simulink model "ARM_Open_loop_simulation"  (R2021a)
settings: Solver=VariableStepAuto  StartTime=0.0  StopTime=50  RelTol=1e-3  EnableMultiTasking=on
StartFcn:
  | clear all
libraries: simulink x1, realtime_pacer_lib x1
settings Model: Creator=johnh  LastModifiedBy=Andy
settings SolverCC: AlgebraicLoopSolver=TrustRegion
settings DataIOCC: ReturnWorkspaceOutputs=off
settings OptimizationCC: LifeSpan=inf
settings DebuggingCC: SFUnexpectedBacktrackingDiag=warning  SFNoUnconditionalDefaultTransitionDiag=warning  SFMachineParentedDataDiag=warning  ArithmeticOperatorsInVariantConditions=warning
settings SFSimCC: SimUseLocalCustomCode=off  CustomCodeUndefinedFunction=UseInterfaceOnly
settings RTWCC: RTWUseLocalCustomCode=off
settings CodeAppCC: StateflowObjectComments=on
settings GRTTargetCC: TargetLangStandard=C89/C90 (ANSI)
settings ConfigComp: CovMetricSettings=dw  CovSaveCumulativeToWorkspaceVar=on  CovSaveSingleToWorkspaceVar=on  CovExternalEMLEnable=off

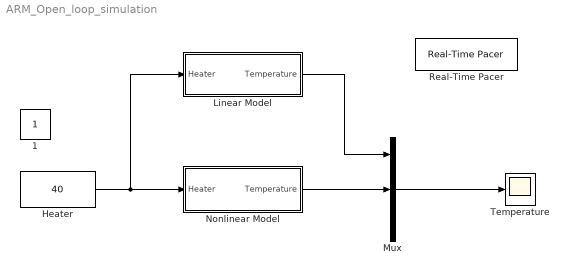
== system ARM_Open_loop_simulation ==
  Heater : simulink/Math Operations/Slider Gain  gain=40  low=0  high=100
  Linear Model : Subsystem
  Mux : Mux  Inputs=3
  Nonlinear Model : Subsystem
  Real-Time Pacer : realtime_pacer_lib/Real-Time Pacer  simTimePerRealTime=1
  Temperature : Scope
  1 : Constant  IOType=siggen
  wires:
  Mux/1 -> Temperature/1
  Linear Model/1(Temperature) -> Mux/1
  Nonlinear Model/1(Temperature) -> Mux/2
  Heater/1 -> Linear Model/1(Heater), Nonlinear Model/1(Heater)

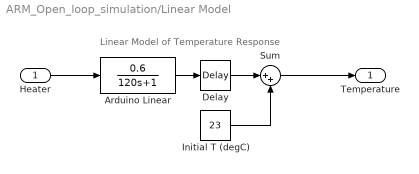
== system ARM_Open_loop_simulation/Linear Model ==
  note: Linear Model of Temperature Response
  Heater : Inport
  Arduino Linear : TransferFcn  Numerator=[0.6]  Denominator=[120 1]
  Delay : TransportDelay  DelayTime=3
  Initial T (degC) : Constant  Value=23
  Sum : Sum  Inputs=|++
  Temperature : Outport
  wires:
  Arduino Linear/1 -> Delay/1
  Delay/1 -> Sum/1
  Initial T (degC)/1 -> Sum/2
  Sum/1 -> Temperature/1
  Heater/1 -> Arduino Linear/1

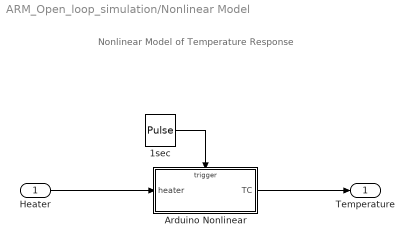
== system ARM_Open_loop_simulation/Nonlinear Model ==
  note: Nonlinear Model of Temperature Response
  Heater : Inport
  1sec : DiscretePulseGenerator  PulseType=Time based  Period=1  PulseWidth=50
  Arduino Nonlinear : Subsystem  TreatAsAtomicUnit=on
  Temperature : Outport
  wires:
  1sec/1 -> Arduino Nonlinear/Trigger
  Arduino Nonlinear/1(TC) -> Temperature/1
  Heater/1 -> Arduino Nonlinear/1(heater)

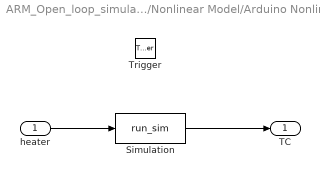
== system ARM_Open_loop_simulation/Nonlinear Model/Arduino Nonlinear ==
  heater : Inport
  Trigger : TriggerPort  VariantControl=Variant
  Simulation : MATLABFcn  MATLABFcn=run_sim
  TC : Outport  InitialOutput=23
  wires:
  heater/1 -> Simulation/1
  Simulation/1 -> TC/1
